simulink model "HydBrakeCU_ESP"  (Simulink 7.9)
settings: Solver=ode45  StartTime=0.0  StopTime=inf  RelTol=1e-3
PreLoadFcn:
  | HydBrakeCU_ESP_params
undefined symbols (not defined in the file or in its folder): Area_Front, Area_Rear, ay_max_off, ay_max_on, ay_per_mu_max_off, ay_per_mu_max_on, Brake_ratio, brake_valve_ctrl_kP, cat1mode1_higher, cat1mode1_lower, cat1mode2_higher, cat1mode2_lower, cat1mode3_higher, cat1mode3_lower, cat2mode1_higher, cat2mode1_lower, cat2mode2_higher, cat2mode2_lower, cat2mode3_higher, cat2mode3_lower, delta_vel, diff_lock_fac, diff_lock_off, diff_lock_on, ESP_ctrl_kD, ESP_ctrl_kI, ESP_ctrl_kP, ESP_ctrl_restore_kI, ESP_min_throttle_fac, f_ax, f_slip, g, higherlimit_highvel, higherlimit_lowvel, highervel_fac, highervelocity_fac, InitialConditionForIntegrator, limit_acc, limit_selectlow, limit_starting, limit_vdiff, locktime_throttle, lowerlimit_highvel, lowerlimit_lowvel, lowervel_fac, lowervelocity_fac, min_throttle, MPS2KMPH, MSR_ctrl_kD, MSR_ctrl_kI, MSR_ctrl_kP, MSR_min_throttle_fac, PID_kP_sideslip, PID_kP_yawrate, RADpS2RpM, rBrake, RpM2RADpS, SH_SL_switch, sideslip_vel_corr, sidesplip_deviation_max ... (+33)
libraries: CarMaker4SL x136, simulink x49, simulink_extras x6
(part 2 of 5)

== system HydBrakeCU_ESP/CarMaker/IPG Vehicle/CarAndTrailer/Forces/Tires ==
  note: The TireXX_Out signals will only be used if FileIdent is "CarMaker-Tire-CM4SL" in the tire parameter file!
      | An example parameter file can be found in Data/Tire/DT_CM4SL_UserTire.
  Sync_In : Inport
  TireFL_In : Inport  Port=2
  TireFR_In : Inport  Port=3
  TireRL_In : Inport  Port=4
  TireRR_In : Inport  Port=5
  Bus Creator{1..4} (4 alike) : BusCreator  Inputs=11
  Demux{1..3,8} (4 alike) : Demux  Outputs=7
  TireFL : Subsystem
  TireFR : Subsystem
  TireRL : Subsystem
  TireRR : Subsystem
  TireFL_Out : Outport
  TireFR_Out : Outport  Port=2
  TireRL_Out : Outport  Port=3
  TireRR_Out : Outport  Port=4
  wires:
  Sync_In/1 -> TireRR/1(Sync_In), TireRL/1(Sync_In), TireFR/1(Sync_In), TireFL/1(Sync_In)
  Bus Creator4/1 -> TireRR_Out/1
  Bus Creator2/1 -> TireRL_Out/1
  Bus Creator1/1 -> TireFR_Out/1
  Demux3/5 -> TireRR/6(Rim_turnv)  "Tire_In Rim_turnv"
  Demux3/4 -> TireRR/5(Rim_rotv)  "Tire_In Rim_rotv"
  Demux3/1 -> TireRR/2(Load)  "Tire_In Load"
  Demux3/7 -> TireRR/8(muRoad)  "Tire_In mu"
  Demux3/6 -> TireRR/7(InclinAngle)  "Tire_In Camber"
  Demux3/2 -> TireRR/3(vxtrans)  "Tire_In vxtrans"
  Demux3/3 -> TireRR/4(vytrans)  "Tire_In vytrans"
  TireRR/11(AlignTrq) -> Bus Creator4/11  "Tire_Out AlignTrq"
  TireRR/10(RollResist) -> Bus Creator4/10  "Tire_Out RollResist"
  TireRR/9(OverturnTrq) -> Bus Creator4/9  "Tire_Out OverturnTrq"
  TireRR/8(LoadFrc) -> Bus Creator4/8  "Tire_Out LoadFrc"
  TireRR/7(SideFrc) -> Bus Creator4/7  "Tire_Out SideFrc"
  TireRR/6(LongFrc) -> Bus Creator4/6  "Tire_Out LongFrc"
  TireRR/5(vBelt) -> Bus Creator4/5  "Tire_Out vBelt"
  TireRR/4(rBelt_eff) -> Bus Creator4/4  "Tire_Out rBelt_eff"
  TireRR/3(TurnSlp) -> Bus Creator4/3  "Tire_Out TurnSlp"
  TireRR/1(Slp) -> Bus Creator4/1  "Tire_Out Slp"
  TireRR/2(Alpha) -> Bus Creator4/2  "Tire_Out Alpha"
  Demux2/5 -> TireRL/6(Rim_turnv)  "Tire_In Rim_turnv"
  Demux2/4 -> TireRL/5(Rim_rotv)  "Tire_In Rim_rotv"
  Demux2/1 -> TireRL/2(Load)  "Tire_In Load"
  Demux2/7 -> TireRL/8(muRoad)  "Tire_In mu"
  Demux2/6 -> TireRL/7(InclinAngle)  "Tire_In Camber"
  Demux2/2 -> TireRL/3(vxtrans)  "Tire_In vxtrans"
  Demux2/3 -> TireRL/4(vytrans)  "Tire_In vytrans"
  TireRL/11(AlignTrq) -> Bus Creator2/11  "Tire_Out AlignTrq"
  TireRL/10(RollResist) -> Bus Creator2/10  "Tire_Out RollResist"
  TireRL/9(OverturnTrq) -> Bus Creator2/9  "Tire_Out OverturnTrq"
  TireRL/8(LoadFrc) -> Bus Creator2/8  "Tire_Out LoadFrc"
  TireRL/7(SideFrc) -> Bus Creator2/7  "Tire_Out SideFrc"
  TireRL/6(LongFrc) -> Bus Creator2/6  "Tire_Out LongFrc"
  TireRL/5(vBelt) -> Bus Creator2/5  "Tire_Out vBelt"
  TireRL/4(rBelt_eff) -> Bus Creator2/4  "Tire_Out rBelt_eff"
  TireRL/3(TurnSlp) -> Bus Creator2/3  "Tire_Out TurnSlp"
  TireRL/1(Slp) -> Bus Creator2/1  "Tire_Out Slp"
  TireRL/2(Alpha) -> Bus Creator2/2  "Tire_Out Alpha"
  Demux1/5 -> TireFR/6(Rim_turnv)  "Tire_In Rim_turnv"
  Demux1/4 -> TireFR/5(Rim_rotv)  "Tire_In Rim_rotv"
  Demux1/1 -> TireFR/2(Load)  "Tire_In Load"
  Demux1/7 -> TireFR/8(muRoad)  "Tire_In mu"
  Demux1/6 -> TireFR/7(InclinAngle)  "Tire_In Camber"
  Demux1/2 -> TireFR/3(vxtrans)  "Tire_In vxtrans"
  Demux1/3 -> TireFR/4(vytrans)  "Tire_In vytrans"
  TireFR/11(AlignTrq) -> Bus Creator1/11  "Tire_Out AlignTrq"
  TireFR/10(RollResist) -> Bus Creator1/10  "Tire_Out RollResist"
  TireFR/9(OverturnTrq) -> Bus Creator1/9  "Tire_Out OverturnTrq"
  TireFR/8(LoadFrc) -> Bus Creator1/8  "Tire_Out LoadFrc"
  TireFR/7(SideFrc) -> Bus Creator1/7  "Tire_Out SideFrc"
  TireFR/6(LongFrc) -> Bus Creator1/6  "Tire_Out LongFrc"
  TireFR/5(vBelt) -> Bus Creator1/5  "Tire_Out vBelt"
  TireFR/4(rBelt_eff) -> Bus Creator1/4  "Tire_Out rBelt_eff"
  TireFR/3(TurnSlp) -> Bus Creator1/3  "Tire_Out TurnSlp"
  TireFR/1(Slp) -> Bus Creator1/1  "Tire_Out Slp"
  TireFR/2(Alpha) -> Bus Creator1/2  "Tire_Out Alpha"
  Demux8/5 -> TireFL/6(Rim_turnv)  "Tire_In Rim_turnv"
  Demux8/4 -> TireFL/5(Rim_rotv)  "Tire_In Rim_rotv"
  TireFL_In/1 -> Demux8/1
  Demux8/1 -> TireFL/2(Load)  "Tire_In Load"
  Demux8/7 -> TireFL/8(muRoad)  "Tire_In mu"
  Demux8/6 -> TireFL/7(InclinAngle)  "Tire_In Camber"
  Demux8/2 -> TireFL/3(vxtrans)  "Tire_In vxtrans"
  Demux8/3 -> TireFL/4(vytrans)  "Tire_In vytrans"
  TireFL/11(AlignTrq) -> Bus Creator3/11  "Tire_Out AlignTrq"
  TireFL/10(RollResist) -> Bus Creator3/10  "Tire_Out RollResist"
  TireFL/9(OverturnTrq) -> Bus Creator3/9  "Tire_Out OverturnTrq"
  TireFL/8(LoadFrc) -> Bus Creator3/8  "Tire_Out LoadFrc"
  TireFL/7(SideFrc) -> Bus Creator3/7  "Tire_Out SideFrc"
  TireFL/6(LongFrc) -> Bus Creator3/6  "Tire_Out LongFrc"
  TireFL/5(vBelt) -> Bus Creator3/5  "Tire_Out vBelt"
  TireFL/4(rBelt_eff) -> Bus Creator3/4  "Tire_Out rBelt_eff"
  TireFL/3(TurnSlp) -> Bus Creator3/3  "Tire_Out TurnSlp"
  TireFL/1(Slp) -> Bus Creator3/1  "Tire_Out Slp"
  TireFL/2(Alpha) -> Bus Creator3/2  "Tire_Out Alpha"
  Bus Creator3/1 -> TireFL_Out/1
  TireFR_In/1 -> Demux1/1
  TireRL_In/1 -> Demux2/1
  TireRR_In/1 -> Demux3/1

== system HydBrakeCU_ESP/CarMaker/IPG Vehicle/CarAndTrailer/Forces/Vehicle Forces ==
  Sync_In : Inport
  Bus Creator1 : BusCreator  Inputs=12
  Bus Creator8 : BusCreator  Inputs=16
  BusCreator1 : BusCreator
  BusCreator2 : BusCreator  Inputs=9
  Demux : Demux  Outputs=16
  Demux1 : Demux  Outputs=12
  Demux2 : Demux  Outputs=13
  Forces : S-Function  FunctionName=CM_Sfun  Parameters='Forces'  EnableBusSupport=off
  Terminator : Terminator
  Sync_Out : Outport
  Car.Virtual : Outport  Port=2
  Car.Aero : Outport  Port=3
  Car.Load : Outport  Port=4
  wires:
  BusCreator1/1 -> Terminator/1  "Aero IF (in)"
  Demux2/13 -> BusCreator2/9  "car Aero Trq_1 z"
  Demux2/12 -> BusCreator2/8  "car Aero Trq_1 y"
  Demux2/11 -> BusCreator2/7  "car Aero Trq_1 x"
  Demux2/10 -> BusCreator2/6  "car Aero Frc_1 z"
  Demux2/9 -> BusCreator2/5  "car Aero Frc_1 y"
  Demux2/8 -> BusCreator2/4  "car Aero Frc_1 x"
  Demux2/7 -> BusCreator2/3  "car Aero PoA_1 z"
  Demux2/6 -> BusCreator2/2  "car Aero PoA_1 y"
  Demux2/5 -> BusCreator2/1  "car Aero PoA_1 x"
  Demux2/4 -> BusCreator1/4  "car Aero tau_1"
  Demux2/3 -> BusCreator1/3  "car Aero ApproachVel_1 z"
  Demux2/2 -> BusCreator1/2  "car Aero ApproachVel_1 y"
  Demux2/1 -> BusCreator1/1  "car Aero ApproachVel_1 x"
  Demux/16 -> Bus Creator8/16  "Car Load_3 tz"
  Demux/15 -> Bus Creator8/15  "Car Load_3 ty"
  Demux/14 -> Bus Creator8/14  "Car Load_3 tx"
  Demux/13 -> Bus Creator8/13  "Car Load_3 mass"
  Demux1/12 -> Bus Creator1/12  "Car Virtual Trq_0 z"
  Demux1/11 -> Bus Creator1/11  "Car Virtual Trq_0 y"
  Demux1/10 -> Bus Creator1/10  "Car Virtual Trq_0 x"
  Demux1/9 -> Bus Creator1/9  "Car Virtual Trq_1 z"
  Demux1/8 -> Bus Creator1/8  "Car Virtual Trq_1 y"
  Demux1/7 -> Bus Creator1/7  "Car Virtual Trq_1 x"
  Demux1/6 -> Bus Creator1/6  "Car Virtual Frc_0 z"
  Demux1/5 -> Bus Creator1/5  "Car Virtual Frc_0 y"
  Demux1/4 -> Bus Creator1/4  "Car Virtual Frc_0 x"
  Sync_In/1 -> Forces/1
  Forces/1 -> Sync_Out/1
  BusCreator2/1 -> Car.Aero/1
  Demux1/1 -> Bus Creator1/1  "Car Virtual Frc_1 x"
  Demux1/2 -> Bus Creator1/2  "Car Virtual Frc_1 y"
  Demux1/3 -> Bus Creator1/3  "Car Virtual Frc_1 z"
  Forces/3 -> Demux2/1
  Forces/2 -> Demux1/1
  Bus Creator1/1 -> Car.Virtual/1
  Bus Creator8/1 -> Car.Load/1
  Demux/1 -> Bus Creator8/1  "Car Load_0 mass"
  Demux/2 -> Bus Creator8/2  "Car Load_0 tx"
  Demux/3 -> Bus Creator8/3  "Car Load_0 ty"
  Demux/4 -> Bus Creator8/4  "Car Load_0 tz"
  Demux/5 -> Bus Creator8/5  "Car Load_1 mass"
  Demux/6 -> Bus Creator8/6  "Car Load_1 tx"
  Demux/7 -> Bus Creator8/7  "Car Load_1 ty"
  Demux/8 -> Bus Creator8/8  "Car Load_1 tz"
  Demux/9 -> Bus Creator8/9  "Car Load_2 mass"
  Demux/10 -> Bus Creator8/10  "Car Load_2 tx"
  Demux/11 -> Bus Creator8/11  "Car Load_2 ty"
  Demux/12 -> Bus Creator8/12  "Car Load_2 tz"
  Forces/4 -> Demux/1

== system HydBrakeCU_ESP/CarMaker/IPG Vehicle/CarAndTrailer/Trailer/CreateBus Car.Hitch.FrcTrq ==
  In1 : Inport
  Bus Creator7 : BusCreator  Inputs=6
  Demux7 : Demux  Outputs=6
  Out1 : Outport
  wires:
  In1/1 -> Demux7/1
  Bus Creator7/1 -> Out1/1
  Demux7/6 -> Bus Creator7/6  "Car Hitch Trq2Car z"
  Demux7/5 -> Bus Creator7/5  "Car Hitch Trq2Car y"
  Demux7/4 -> Bus Creator7/4  "Car Hitch Trq2Car x"
  Demux7/3 -> Bus Creator7/3  "Car Hitch Frc2Car z"
  Demux7/2 -> Bus Creator7/2  "Car Hitch Frc2Car y"
  Demux7/1 -> Bus Creator7/1  "Car Hitch Frc2Car x"

== system HydBrakeCU_ESP/CarMaker/IPG Vehicle/CarAndTrailer/Trailer/CreateBus Vhcl.Motion ==
  In1 : Inport
  BusCreator : BusCreator  Inputs=15
  Demux : Demux  Outputs=15
  Out1 : Outport
  wires:
  Demux/15 -> BusCreator/15  "Vhcl YawAcc"
  Demux/14 -> BusCreator/14  "Vhcl YawVel"
  Demux/13 -> BusCreator/13  "Vhcl Yaw"
  Demux/12 -> BusCreator/12  "Vhcl PitchAcc"
  Demux/11 -> BusCreator/11  "Vhcl PitchVel"
  Demux/10 -> BusCreator/10  "Vhcl Pitch"
  Demux/9 -> BusCreator/9  "Vhcl RollAcc"
  Demux/8 -> BusCreator/8  "Vhcl RollVel"
  Demux/7 -> BusCreator/7  "Vhcl Roll"
  Demux/6 -> BusCreator/6  "Vhcl Hitch_Pos z"
  Demux/5 -> BusCreator/5  "Vhcl Hitch_Pos y"
  Demux/4 -> BusCreator/4  "Vhcl Hitch_Pos x"
  Demux/3 -> BusCreator/3  "Vhcl sRoad"
  Demux/2 -> BusCreator/2  "Vhcl Distance"
  Demux/1 -> BusCreator/1  "Vhcl v"
  In1/1 -> Demux/1
  BusCreator/1 -> Out1/1

== system HydBrakeCU_ESP/CarMaker/IPG Vehicle/CarAndTrailer/Trailer/CreateBus Vhcl.PoI ==
  In1 : Inport
  Bus Creator3 : BusCreator  Inputs=18
  Demux3 : Demux  Outputs=18
  Out1 : Outport
  wires:
  Demux3/18 -> Bus Creator3/18  "Vhcl PoI_GCS Elev"
  Demux3/17 -> Bus Creator3/17  "Vhcl PoI_GCS Lat"
  Demux3/16 -> Bus Creator3/16  "Vhcl PoI_GCS Long"
  Demux3/15 -> Bus Creator3/15  "Vhcl PoI_Acc_1 z"
  Demux3/14 -> Bus Creator3/14  "Vhcl PoI_Acc_1 y"
  Demux3/13 -> Bus Creator3/13  "Vhcl PoI_Acc_1 x"
  Demux3/12 -> Bus Creator3/12  "Vhcl PoI_Vel_1 z"
  Demux3/11 -> Bus Creator3/11  "Vhcl PoI_Vel_1 y"
  Demux3/10 -> Bus Creator3/10  "Vhcl PoI_Vel_1 x"
  Demux3/9 -> Bus Creator3/9  "Vhcl PoI_Acc z"
  Demux3/8 -> Bus Creator3/8  "Vhcl PoI_Acc y"
  Demux3/7 -> Bus Creator3/7  "Vhcl PoI_Acc x"
  Demux3/6 -> Bus Creator3/6  "Vhcl PoI_Vel z"
  Demux3/5 -> Bus Creator3/5  "Vhcl PoI_Vel y"
  Demux3/4 -> Bus Creator3/4  "Vhcl PoI_Vel x"
  Demux3/3 -> Bus Creator3/3  "Vhcl PoI_Pos z"
  Demux3/2 -> Bus Creator3/2  "Vhcl PoI_Pos y"
  In1/1 -> Demux3/1
  Bus Creator3/1 -> Out1/1
  Demux3/1 -> Bus Creator3/1  "Vhcl PoI_Pos x"

== system HydBrakeCU_ESP/CarMaker/IPG Vehicle/CarAndTrailer/Trailer/CreateBus Vhcl.Steering ==
  In1 : Inport
  Bus Creator3 : BusCreator
  Demux : Demux
  Out1 : Outport
  wires:
  Bus Creator3/1 -> Out1/1
  Demux/1 -> Bus Creator3/1  "Vhcl Steering Ang"
  Demux/3 -> Bus Creator3/3  "Vhcl Steering AngAcc"
  Demux/2 -> Bus Creator3/2  "Vhcl Steering AngVel"
  Demux/4 -> Bus Creator3/4  "Vhcl Steering Trq"
  In1/1 -> Demux/1

== system HydBrakeCU_ESP/CarMaker/IPG Vehicle/CarAndTrailer/Trailer/CreateBus Vhcl.Wheel.FL ==
  In1 : Inport
  Bus Creator3 : BusCreator  Inputs=14
  Demux3 : Demux  Outputs=14
  Out1 : Outport
  wires:
  Demux3/14 -> Bus Creator3/14  "Vhcl Wheel FL Trq_WhlBearing"
  Demux3/13 -> Bus Creator3/13  "Vhcl Wheel FL Trq_T2W"
  Demux3/12 -> Bus Creator3/12  "Vhcl Wheel FL SideSlip"
  Demux3/11 -> Bus Creator3/11  "Vhcl Wheel FL LongSlip"
  Demux3/10 -> Bus Creator3/10  "Vhcl Wheel FL vBelt"
  Demux3/9 -> Bus Creator3/9  "Vhcl Wheel FL Fz"
  Demux3/8 -> Bus Creator3/8  "Vhcl Wheel FL Fy"
  Demux3/7 -> Bus Creator3/7  "Vhcl Wheel FL Fx"
  Demux3/6 -> Bus Creator3/6  "Vhcl Wheel FL r_zxy z"
  Demux3/5 -> Bus Creator3/5  "Vhcl Wheel FL r_zxy y"
  Demux3/4 -> Bus Creator3/4  "Vhcl Wheel FL r_zxy x"
  Demux3/3 -> Bus Creator3/3  "Vhcl Wheel FL t z"
  Demux3/2 -> Bus Creator3/2  "Vhcl Wheel FL t y"
  In1/1 -> Demux3/1
  Bus Creator3/1 -> Out1/1
  Demux3/1 -> Bus Creator3/1  "Vhcl Wheel FL t x"

== system HydBrakeCU_ESP/CarMaker/IPG Vehicle/CarAndTrailer/Trailer/CreateBus Vhcl.Wheel.FR ==
  In1 : Inport
  Bus Creator3 : BusCreator  Inputs=14
  Demux3 : Demux  Outputs=14
  Out1 : Outport
  wires:
  Demux3/14 -> Bus Creator3/14  "Vhcl Wheel FR Trq_WhlBearing"
  Demux3/13 -> Bus Creator3/13  "Vhcl Wheel FR Trq_T2W"
  Demux3/12 -> Bus Creator3/12  "Vhcl Wheel FR SideSlip"
  Demux3/11 -> Bus Creator3/11  "Vhcl Wheel FR LongSlip"
  Demux3/10 -> Bus Creator3/10  "Vhcl Wheel FR vBelt"
  Demux3/9 -> Bus Creator3/9  "Vhcl Wheel FR Fz"
  Demux3/8 -> Bus Creator3/8  "Vhcl Wheel FR Fy"
  Demux3/7 -> Bus Creator3/7  "Vhcl Wheel FR Fx"
  Demux3/6 -> Bus Creator3/6  "Vhcl Wheel FR r_zxy z"
  Demux3/5 -> Bus Creator3/5  "Vhcl Wheel FR r_zxy y"
  Demux3/4 -> Bus Creator3/4  "Vhcl Wheel FR r_zxy x"
  Demux3/3 -> Bus Creator3/3  "Vhcl Wheel FR t z"
  Demux3/2 -> Bus Creator3/2  "Vhcl Wheel FR t y"
  In1/1 -> Demux3/1
  Bus Creator3/1 -> Out1/1
  Demux3/1 -> Bus Creator3/1  "Vhcl Wheel FR t x"

== system HydBrakeCU_ESP/CarMaker/IPG Vehicle/CarAndTrailer/Trailer/CreateBus Vhcl.Wheel.RL ==
  In1 : Inport
  Bus Creator3 : BusCreator  Inputs=14
  Demux3 : Demux  Outputs=14
  Out1 : Outport
  wires:
  Demux3/14 -> Bus Creator3/14  "Vhcl Wheel RL Trq_WhlBearing"
  Demux3/13 -> Bus Creator3/13  "Vhcl Wheel RL Trq_T2W"
  Demux3/12 -> Bus Creator3/12  "Vhcl Wheel RL SideSlip"
  Demux3/11 -> Bus Creator3/11  "Vhcl Wheel RL LongSlip"
  Demux3/10 -> Bus Creator3/10  "Vhcl Wheel RL vBelt"
  Demux3/9 -> Bus Creator3/9  "Vhcl Wheel RL Fz"
  Demux3/8 -> Bus Creator3/8  "Vhcl Wheel RL Fy"
  Demux3/7 -> Bus Creator3/7  "Vhcl Wheel RL Fx"
  Demux3/6 -> Bus Creator3/6  "Vhcl Wheel RL r_zxy z"
  Demux3/5 -> Bus Creator3/5  "Vhcl Wheel RL r_zxy y"
  Demux3/4 -> Bus Creator3/4  "Vhcl Wheel RL r_zxy x"
  Demux3/3 -> Bus Creator3/3  "Vhcl Wheel RL t z"
  Demux3/2 -> Bus Creator3/2  "Vhcl Wheel RL t y"
  In1/1 -> Demux3/1
  Bus Creator3/1 -> Out1/1
  Demux3/1 -> Bus Creator3/1  "Vhcl Wheel RL t x"

== system HydBrakeCU_ESP/CarMaker/IPG Vehicle/CarAndTrailer/Trailer/CreateBus Vhcl.Wheel.RR ==
  In1 : Inport
  Bus Creator3 : BusCreator  Inputs=14
  Demux3 : Demux  Outputs=14
  Out1 : Outport
  wires:
  Demux3/14 -> Bus Creator3/14  "Vhcl Wheel RR Trq_WhlBearing"
  Demux3/13 -> Bus Creator3/13  "Vhcl Wheel RR Trq_T2W"
  Demux3/12 -> Bus Creator3/12  "Vhcl Wheel RR SideSlip"
  Demux3/11 -> Bus Creator3/11  "Vhcl Wheel RR LongSlip"
  Demux3/10 -> Bus Creator3/10  "Vhcl Wheel RR vBelt"
  Demux3/9 -> Bus Creator3/9  "Vhcl Wheel RR Fz"
  Demux3/8 -> Bus Creator3/8  "Vhcl Wheel RR Fy"
  Demux3/7 -> Bus Creator3/7  "Vhcl Wheel RR Fx"
  Demux3/6 -> Bus Creator3/6  "Vhcl Wheel RR r_zxy z"
  Demux3/5 -> Bus Creator3/5  "Vhcl Wheel RR r_zxy y"
  Demux3/4 -> Bus Creator3/4  "Vhcl Wheel RR r_zxy x"
  Demux3/3 -> Bus Creator3/3  "Vhcl Wheel RR t z"
  Demux3/2 -> Bus Creator3/2  "Vhcl Wheel RR t y"
  In1/1 -> Demux3/1
  Bus Creator3/1 -> Out1/1
  Demux3/1 -> Bus Creator3/1  "Vhcl Wheel RR t x"

== system HydBrakeCU_ESP/CarMaker/IPG Vehicle/Brake/HydBrakeCU Example/ESP Controller/ESP General System ==
  ESP Input Signals : Inport
  User Input Signals : Inport  Port=2
  Vehicle Input Params : Inport  Port=3
  Ideal_In : Inport  Port=4
  ABS : Subsystem
  ASR : Subsystem
  Bus Creator : BusCreator  Inputs=7
  Bus Creator2 : BusCreator  Inputs=5
  Bus Creator3 : BusCreator  Inputs=6
  Bus Creator4 : BusCreator
  ESP : Subsystem
  HSA : Subsystem
  Master Controller : Subsystem
  Signal Handling : Subsystem
  ESP Out : Outport
  wires:
  Bus Creator/1 -> ESP Out/1
  ESP Input Signals/1 -> Signal Handling/1(ESP In)
  ESP/1(ESP On) -> Master Controller/2(ESP On)  "ESP On"
  ESP/2(Pilot Valves) -> Bus Creator2/1  "Pilot Valves"
  ESP/3(Suction Valves) -> Bus Creator2/2  "Suction Valves"
  ESP/4(Brake Valves) -> Bus Creator2/3  "Brake Valves"
  ESP/5(Pump Ctrl) -> Bus Creator2/4  "Pump Ctrl"
  ESP/6(Gas_Out) -> Bus Creator2/5  "Gas_Out"
  Bus Creator2/1 -> Master Controller/3(ESP Bus)  "ESP Bus"
  ASR/1(ASR On) -> Master Controller/4(ASR On)  "ASR On"
  ABS/1(ABS On) -> Master Controller/6(ABS On)  "ABS On"
  Bus Creator3/1 -> Master Controller/5(ASR Bus)  "ASR Bus"
  Master Controller/1(ECU Flags) -> Bus Creator/1  "ECU Flags"
  Master Controller/2(Brake Valves) -> Bus Creator/2  "Brake Valves"
  Master Controller/3(Pilot Valves) -> Bus Creator/3  "Pilot Valves"
  Master Controller/4(Suction Valves) -> Bus Creator/4  "Suction Valves"
  Master Controller/5(Pump Ctrl) -> Bus Creator/5  "Pump Ctrl"
  ASR/2(Pilot Valves) -> Bus Creator3/1  "Pilot Valves"
  ASR/3(Suction Valves) -> Bus Creator3/2  "Suction Valves"
  ASR/4(Brake Valves) -> Bus Creator3/3  "Brake Valves"
  ASR/5(Pump Ctrl) -> Bus Creator3/4  "Pump Ctrl"
  ASR/6(Gas_out) -> Bus Creator3/5  "Gas_Out"
  ABS/2(Pilot Valves) -> Bus Creator4/1  "Pilot Valves"
  ABS/3(Suction Valves) -> Bus Creator4/2  "Suction Valves"
  ABS/4(Brake Valves) -> Bus Creator4/3  "Brake Valves"
  ABS/5(Pump Ctrl) -> Bus Creator4/4  "Pump Ctrl"
  Bus Creator4/1 -> Master Controller/7(ABS Bus)  "ABS Bus"
  User Input Signals/1 -> Master Controller/10(User In), ESP/4(User_In), ASR/4(User_In), ABS/4(User_In)
  Vehicle Input Params/1 -> Signal Handling/2(Vehicle Params), ESP/3(Vehicle Params), ASR/3(Vehicle Params), ABS/3(Vehicle Params)
  ASR/7(Diff_Torque) -> Bus Creator3/6  "Diff_Torque"
  Master Controller/6(Diff_Torque) -> Bus Creator/6  "Diff_Torque"
  Ideal_In/1 -> HSA/2(Ideal_In), ABS/2(Ideal_In), ESP/2(Ideal_In), ASR/2(Ideal_In)
  Master Controller/7(VC_Out) -> Bus Creator/7  "VC_Out"
  Signal Handling/2(Signal Bus ESP) -> ESP/1(ESP Signal Bus)
  Signal Handling/3(Signal Bus ASR) -> ASR/1(ASR Signal Bus)
  Signal Handling/4(Signal Bus ABS) -> ABS/1(ABS Signal Bus)
  Signal Handling/5(Signal Bus HSA) -> HSA/1(HSA Signal Bus)
  HSA/1(HSA On) -> Master Controller/8(HSA On)
  HSA/2(BrakePark_Out) -> Master Controller/9(HSA Bus)  "BrakePark"
  Signal Handling/1(Signal Bus Master Controller) -> Master Controller/1(Signal In)

== system HydBrakeCU_ESP/CarMaker/IPG Vehicle/Brake/HydBrakeCU Example/ESP Controller/ESP Input Signals ==
  HydBrakeCtrl_In : Inport
  " " : simulink_extras/Transformations/Radians to Degrees
  "   " : simulink_extras/Transformations/Radians to Degrees
  Bus Creator1 : BusCreator  Inputs=20
  Bus Selector : BusSelector  OutputSignals=Omega_B z,Acc_B y,Acc_B x
  Bus Selector1 : BusSelector  OutputSignals=HydBrakeCU pMC,HydBrakeCU pWB_FL,HydBrakeCU pWB_FR,HydBrakeCU pWB_RL,HydBrakeCU pWB_RR,HydBrakeCU Park,HydBrakeCU Pedal
  Car InertialSensor : CarMaker4SL/Car InertialSensor  xname=YRS
  Gain{,6,9..10,12..17} (10 alike) : Gain  SaturateOnIntegerOverflow=on  OutDataTypeStr=Inherit: Same as input  ParamDataTypeStr=Inherit: Same as input
  Gain{1..5,11} (6 alike) : Gain  Gain=RADpS2RpM  SaturateOnIntegerOverflow=on  OutDataTypeStr=Inherit: Same as input  ParamDataTypeStr=Inherit: Same as input
  Gain7 : Gain  Gain=1/g  SaturateOnIntegerOverflow=on  OutDataTypeStr=Inherit: Same as input  ParamDataTypeStr=Inherit: Same as input
  Gain8 : Gain  Gain=1/g  SaturateOnIntegerOverflow=on  OutDataTypeStr=Inherit: Same as input  ParamDataTypeStr=Inherit: Same as input
  Read CM Dict1 : CarMaker4SL/Read CM Dict  xname=Car.WheelSpd_FL  xsync=off
  Read CM Dict10 : CarMaker4SL/Read CM Dict  xname=PT.Clutch.rotv_out  xsync=off
  Read CM Dict11 : CarMaker4SL/Read CM Dict  xname=Steer.WhlAng  xsync=off
  Read CM Dict12 : CarMaker4SL/Read CM Dict  xname=PT.Engine.Trq  xsync=off
  Read CM Dict15 : CarMaker4SL/Read CM Dict  xname=PT.GearBox.GearNo  xsync=off
  Read CM Dict2 : CarMaker4SL/Read CM Dict  xname=Car.WheelSpd_FR  xsync=off
  Read CM Dict3 : CarMaker4SL/Read CM Dict  xname=Car.WheelSpd_RL  xsync=off
  Read CM Dict4 : CarMaker4SL/Read CM Dict  xname=Car.WheelSpd_RR  xsync=off
  Read CM Dict7 : CarMaker4SL/Read CM Dict  xname=PT.Engine.rotv  xsync=off
  Read CM Dict9 : CarMaker4SL/Read CM Dict  xname=VC.Gas  xsync=off
  Terminator : Terminator
  ESP Signals : Outport
  wires:
  Gain9/1 -> Bus Creator1/9  "Engine crankshaft output torque [Nm]"
  Gain13/1 -> Bus Creator1/14  "GearState [-]"
  " "/1 -> Bus Creator1/13  "Steering Wheel Angle [deg]"
  Gain11/1 -> Bus Creator1/12  "Torque Converter Speed [rpm]"
  Gain10/1 -> Bus Creator1/10  "Master Cylinder Pressure [bar]"
  Gain8/1 -> Bus Creator1/7  "Sensor Longitudinal acceleration [g]"
  Gain7/1 -> Bus Creator1/6  "Sensor Lateral acceleration [g]"
  "   "/1 -> Bus Creator1/5  "Sensor YawRate [degs]"
  Gain4/1 -> Bus Creator1/4  "WheelSpd RR [rpm]"
  Gain5/1 -> Bus Creator1/3  "WheelSpd RL [rpm]"
  Gain3/1 -> Bus Creator1/2  "WheelSpd FR [rpm]"
  Gain2/1 -> Bus Creator1/1  "WheelSpd FL [rpm]"
  Read CM Dict15/1 -> Gain13/1  "GearNumber [-]"
  Gain1/1 -> Bus Creator1/8  "Engine Speed [rpm]"
  Bus Selector/1 -> "   "/1  "<Omega_B z>"
  Bus Selector/3 -> Gain8/1  "<Acc_B x>"
  Car InertialSensor/2 -> Bus Selector/1
  Read CM Dict11/1 -> " "/1  "Steering Angle [rad]"
  Read CM Dict10/1 -> Gain11/1  "Clucth OutShaft [rad/s]"
  Read CM Dict9/1 -> Gain/1  "Accelerator pedal [-]"
  Bus Selector1/1 -> Gain10/1  "<HydBrakeCU pMC>"
  Read CM Dict1/1 -> Gain2/1  "WheelSpd FL [rad]/s]"
  Read CM Dict2/1 -> Gain3/1  "WheelSpd FR [rad/s]"
  Read CM Dict3/1 -> Gain5/1  "WheelSpd RL [rad/s]"
  Bus Selector/2 -> Gain7/1  "<Acc_B y>"
  Read CM Dict4/1 -> Gain4/1  "WheelSpd RR [rad/s]"
  Gain/1 -> Bus Creator1/11  "Throttle Valve Position"
  Read CM Dict12/1 -> Gain9/1  "Engine Torque [Nm]"
  Read CM Dict7/1 -> Gain1/1  "Engine RotVel [rad/s]"
  Bus Creator1/1 -> ESP Signals/1
  Bus Selector1/5 -> Gain15/1  "<HydBrakeCU pWB_RR>"
  Bus Selector1/4 -> Gain14/1  "<HydBrakeCU pWB_RL>"
  Bus Selector1/3 -> Gain12/1  "<HydBrakeCU pWB_FR>"
  Bus Selector1/2 -> Gain6/1  "<HydBrakeCU pWB_FL>"
  Gain6/1 -> Bus Creator1/15  "Cylinder Pressure FL [bar]"
  Gain12/1 -> Bus Creator1/16  "Cylinder Pressure FR [bar]"
  Gain14/1 -> Bus Creator1/17  "Cylinder Pressure RL [bar]"
  Gain15/1 -> Bus Creator1/18  "Cylinder Pressure RR [bar]"
  HydBrakeCtrl_In/1 -> Bus Selector1/1
  Car InertialSensor/1 -> Terminator/1
  Bus Selector1/6 -> Gain16/1  "<HydBrakeCU Park>"
  Gain16/1 -> Bus Creator1/19  "Park Brake Position"
  Bus Selector1/7 -> Gain17/1  "<HydBrakeCU Pedal>"
  Gain17/1 -> Bus Creator1/20  "Brake Pedal Position"

== system HydBrakeCU_ESP/CarMaker/IPG Vehicle/Brake/HydBrakeCU Example/ESP Controller/Ideal Input Signals ==
  Bus Creator1 : BusCreator  Inputs=8
  Bus Creator2 : BusCreator
  Bus Creator3 : BusCreator  Inputs=2
  Bus Creator4 : BusCreator  Inputs=2
  Bus Creator5 : BusCreator  Inputs=3
  Bus Creator6 : BusCreator  Inputs=2
  Read CM Dict1 : CarMaker4SL/Read CM Dict  xname=Car.Pitch  xsync=off
  Read CM Dict10 : CarMaker4SL/Read CM Dict  xname=Car.FzRL  xsync=off
  Read CM Dict11 : CarMaker4SL/Read CM Dict  xname=Car.YawRate  xsync=off
  Read CM Dict13 : CarMaker4SL/Read CM Dict  xname=Car.CRL.Trq_T2W  xsync=off
  Read CM Dict14 : CarMaker4SL/Read CM Dict  xname=Car.LongSlipRL  xsync=off
  Read CM Dict16 : CarMaker4SL/Read CM Dict  xname=Car.CRR.Trq_T2W  xsync=off
  Read CM Dict17 : CarMaker4SL/Read CM Dict  xname=Car.FzRR  xsync=off
  Read CM Dict19 : CarMaker4SL/Read CM Dict  xname=Car.LongSlipRR  xsync=off
  Read CM Dict2 : CarMaker4SL/Read CM Dict  xname=Car.v  xsync=off
  Read CM Dict3 : CarMaker4SL/Read CM Dict  xname=Car.muRoadFR  xsync=off
  Read CM Dict4 : CarMaker4SL/Read CM Dict  xname=Car.muRoadRL  xsync=off
  Read CM Dict5 : CarMaker4SL/Read CM Dict  xname=Car.SideSlipAngle  xsync=off
  Read CM Dict6 : CarMaker4SL/Read CM Dict  xname=Car.muRoadFL  xsync=off
  Read CM Dict7 : CarMaker4SL/Read CM Dict  xname=Car.muRoadRR  xsync=off
  Read CM Dict8 : CarMaker4SL/Read CM Dict  xname=Car.vx  xsync=off
  Read CM Dict9 : CarMaker4SL/Read CM Dict  xname=Car.vy  xsync=off
  Ideal_In : Outport
  wires:
  Read CM Dict17/1 -> Bus Creator4/2  "Ideal_FzRR"
  Read CM Dict10/1 -> Bus Creator4/1  "Ideal_FzRL"
  Read CM Dict16/1 -> Bus Creator3/2  "Ideal_Trq2WRR"
  Read CM Dict13/1 -> Bus Creator3/1  "Ideal_Trq2WRL"
  Read CM Dict6/1 -> Bus Creator2/1  "Ideal_muFL"
  Read CM Dict3/1 -> Bus Creator2/2  "Ideal_muFR"
  Read CM Dict4/1 -> Bus Creator2/3  "Ideal_muRL"
  Read CM Dict7/1 -> Bus Creator2/4  "Ideal_muRR"
  Bus Creator1/1 -> Ideal_In/1
  Read CM Dict1/1 -> Bus Creator1/1  "Ideal_Pitch"
  Read CM Dict5/1 -> Bus Creator1/3  "Ideal_SideSlipAngle"
  Read CM Dict2/1 -> Bus Creator5/1  "Ideal_Velocity"
  Read CM Dict8/1 -> Bus Creator5/2  "Ideal_Velocity_x"
  Bus Creator5/1 -> Bus Creator1/2  "Ideal_Velocity"
  Read CM Dict9/1 -> Bus Creator5/3  "Ideal_Velocity_y"
  Read CM Dict14/1 -> Bus Creator6/1  "Ideal_SlipRL"
  Read CM Dict19/1 -> Bus Creator6/2  "Ideal_SlipRR"
  Read CM Dict11/1 -> Bus Creator1/4  "Ideal_YawRate"
  Bus Creator2/1 -> Bus Creator1/5  "Ideal_mu"
  Bus Creator3/1 -> Bus Creator1/6  "Idea_Trq2W"
  Bus Creator4/1 -> Bus Creator1/7  "Ideal_Fz"
  Bus Creator6/1 -> Bus Creator1/8  "Ideal_Slip"

== system HydBrakeCU_ESP/CarMaker/IPG Vehicle/Brake/HydBrakeCU Example/ESP Controller/Output Signals ESP ==
  ESP Out : Inport
  Bus Creator : BusCreator  Inputs=6
  Bus Selector : BusSelector  OutputSignals=ECU Flags,Brake Valves,Pilot Valves,Suction Valves,Pump Ctrl,VC_Out.BrakePark,VC_Out.Brake Pedal Position,Diff_Torque,VC_Out.Load_lim
  Bus Selector1 : BusSelector  OutputSignals=ESP On,ASR On,ABS On,HSA On
  Bus Selector2 : BusSelector  OutputSignals=ASR On,MSR On,BMR On
  Bus Selector4 : BusSelector  OutputSignals=FrontDiff_Torque
  Data Type Conversion : DataTypeConversion
  Define CM Dict1 : CarMaker4SL/Define CM Dict  xname=ESP.ASR.MSR.active  xmono=off  xtype=Char  xdvaplace=VC  xnstates=2  xfirststate=0  xinitial=0
  Define CM Dict10 : CarMaker4SL/Define CM Dict  xname=ESP.ESP.active  xmono=off  xtype=Char  xdvaplace=VC  xnstates=2  xfirststate=0  xinitial=0
  Define CM Dict2 : CarMaker4SL/Define CM Dict  xname=ESP.ASR.BMR.active  xmono=off  xtype=Char  xdvaplace=VC  xnstates=2  xfirststate=0  xinitial=0
  Define CM Dict3 : CarMaker4SL/Define CM Dict  xname=ESP.ASR.active  xmono=off  xtype=Char  xdvaplace=VC  xnstates=2  xfirststate=0  xinitial=0
  Define CM Dict4 : CarMaker4SL/Define CM Dict  xname=ESP.HSA.active  xmono=off  xtype=Char  xdvaplace=VC  xnstates=2  xfirststate=0  xinitial=0
  Define CM Dict6 : CarMaker4SL/Define CM Dict  xname=ESP.ESP.lamp  xmono=off  xtype=Char  xdvaplace=VC  xnstates=2  xfirststate=0  xinitial=0
  Define CM Dict9 : CarMaker4SL/Define CM Dict  xname=ESP.ABS.Active  xmono=off  xtype=Char  xdvaplace=VC  xnstates=2  xfirststate=0  xinitial=0
  Logical Operator : Logic  Operator=OR  AllPortsSameDT=off  OutDataTypeStr=boolean
  Read CM Dict3 : CarMaker4SL/Read CM Dict  xname=ESP.User.ESP_off  xsync=off
  Write CM Dict : CarMaker4SL/Write CM Dict  xname=PT.ECU.Load_lim  xsync=off
  Write CM Dict12 : CarMaker4SL/Write CM Dict  xname=ESP.ASR.MSR.active  xsync=off
  Write CM Dict13 : CarMaker4SL/Write CM Dict  xname=ESP.ASR.BMR.active  xsync=off
  Write CM Dict15 : CarMaker4SL/Write CM Dict  xname=ESP.ASR.active  xsync=off
  Write CM Dict17 : CarMaker4SL/Write CM Dict  xname=ESP.ABS.Active  xsync=off
  Write CM Dict18 : CarMaker4SL/Write CM Dict  xname=ESP.ESP.active  xsync=off
  Write CM Dict19 : CarMaker4SL/Write CM Dict  xname=PT.Gen.DL.FDiff.DVA.Trq_A2B  xsync=off
  Write CM Dict20 : CarMaker4SL/Write CM Dict  xname=ESP.HSA.active  xsync=off
  Write CM Dict21 : CarMaker4SL/Write CM Dict  xname=ESP.ESP.lamp  xsync=off
  HydBrakeCU_Out : Outport
  wires:
  ESP Out/1 -> Bus Selector/1
  Bus Selector/1 -> Bus Selector1/1  "<ECU Flags>"
  Bus Selector1/2 -> Bus Selector2/1  "<ASR On>"
  Bus Selector1/1 -> Logical Operator/2, Write CM Dict18/1  "<ESP On>"
  Bus Selector1/3 -> Write CM Dict17/1  "<ABS On>"
  Bus Selector2/1 -> Write CM Dict15/1  "<ASR On>"
  Bus Selector2/2 -> Write CM Dict12/1  "<MSR On>"
  Bus Selector2/3 -> Write CM Dict13/1  "<BMR On>"
  Bus Selector4/1 -> Write CM Dict19/1  "<FrontDiff_Torque>"
  Bus Selector/8 -> Bus Selector4/1  "<Diff_Torque>"
  Bus Selector1/4 -> Write CM Dict20/1  "<HSA On>"
  Logical Operator/1 -> Data Type Conversion/1
  Read CM Dict3/1 -> Logical Operator/1
  Data Type Conversion/1 -> Write CM Dict21/1
  Bus Selector/2 -> Bus Creator/1  "<Brake Valves>"
  Bus Selector/3 -> Bus Creator/2  "<Pilot Valves>"
  Bus Selector/4 -> Bus Creator/3  "<Suction Valves>"
  Bus Selector/5 -> Bus Creator/4  "<Pump Ctrl>"
  Bus Creator/1 -> HydBrakeCU_Out/1
  Bus Selector/6 -> Bus Creator/5  "<BrakePark>"
  Bus Selector/9 -> Write CM Dict/1  "<Load_lim>"
  Bus Selector/7 -> Bus Creator/6  "<Brake Pedal Position>"

== system HydBrakeCU_ESP/CarMaker/IPG Vehicle/Brake/HydBrakeCU Example/ESP Controller/User Input Signals1 ==
  note: User_Drive: 1 = Front; 2 = Rear; 3 = AllWheel
  Bus Creator1 : BusCreator  Inputs=5
  Bus Creator2 : BusCreator  Inputs=5
  Bus Creator3 : BusCreator  Inputs=2
  Bus Creator4 : BusCreator  Inputs=2
  Define CM Dict1 : CarMaker4SL/Define CM Dict  xname=ESP.User.ESP_off  xmono=off  xtype=Char  xdvaplace=IO_Out  xnstates=2  xfirststate=0  xinitial=0
  Define CM Dict10 : CarMaker4SL/Define CM Dict  xname=ESP.User.HSA_off  xmono=off  xtype=Char  xdvaplace=IO_Out  xnstates=2  xfirststate=0  xinitial=0
  Define CM Dict11 : CarMaker4SL/Define CM Dict  xname=ESP.User.oneWheel_on  xmono=off  xtype=Char  xdvaplace=IO_Out  xnstates=2  xfirststate=0  xinitial=0
  Define CM Dict2 : CarMaker4SL/Define CM Dict  xname=ESP.User.ASR_off  xmono=off  xtype=Char  xdvaplace=IO_Out  xnstates=2  xfirststate=0  xinitial=0
  Define CM Dict3 : CarMaker4SL/Define CM Dict  xname=ESP.User.ABS_off  xmono=off  xtype=Char  xdvaplace=IO_Out  xnstates=2  xfirststate=0  xinitial=0
  Define CM Dict4 : CarMaker4SL/Define CM Dict  xname=ESP.User.ESP_all_off  xmono=off  xtype=Char  xdvaplace=IO_Out  xnstates=2  xfirststate=0  xinitial=0
  Define CM Dict5 : CarMaker4SL/Define CM Dict  xname=ESP.User.Drive  xmono=off  xtype=Char  xdvaplace=IO_Out  xnstates=3  xfirststate=1  xinitial=1
  Define CM Dict6 : CarMaker4SL/Define CM Dict  xname=ESP.User.SideSlip_estimator_on  xmono=off  xtype=Char  xdvaplace=IO_Out  xnstates=2  xfirststate=0  xinitial=0
  Define CM Dict7 : CarMaker4SL/Define CM Dict  xname=ESP.User.mue_estimator_on  xmono=off  xtype=Char  xdvaplace=IO_Out  xnstates=2  xfirststate=0  xinitial=0
  Define CM Dict8 : CarMaker4SL/Define CM Dict  xname=ESP.User.DiffLockDVA_on  xmono=off  xtype=Char  xdvaplace=IO_Out  xnstates=2  xfirststate=0  xinitial=0
  Define CM Dict9 : CarMaker4SL/Define CM Dict  xname=ESP.User.DiffLockDVA_Trq  xunit=Nm  xmono=off  xtype=Double4  xdvaplace=IO_Out  xnstates=2  xfirststate=0  xinitial=0
  Read CM Dict1 : CarMaker4SL/Read CM Dict  xname=ESP.User.Drive  xsync=off
  Read CM Dict10 : CarMaker4SL/Read CM Dict  xname=ESP.User.HSA_off  xsync=off
  Read CM Dict11 : CarMaker4SL/Read CM Dict  xname=ESP.User.oneWheel_on  xsync=off
  Read CM Dict2 : CarMaker4SL/Read CM Dict  xname=ESP.User.ESP_all_off  xsync=off
  Read CM Dict3 : CarMaker4SL/Read CM Dict  xname=ESP.User.ESP_off  xsync=off
  Read CM Dict4 : CarMaker4SL/Read CM Dict  xname=ESP.User.ASR_off  xsync=off
  Read CM Dict5 : CarMaker4SL/Read CM Dict  xname=ESP.User.ABS_off  xsync=off
  Read CM Dict6 : CarMaker4SL/Read CM Dict  xname=ESP.User.SideSlip_estimator_on  xsync=off
  Read CM Dict7 : CarMaker4SL/Read CM Dict  xname=ESP.User.mue_estimator_on  xsync=off
  Read CM Dict8 : CarMaker4SL/Read CM Dict  xname=ESP.User.DiffLockDVA_on  xsync=off
  Read CM Dict9 : CarMaker4SL/Read CM Dict  xname=ESP.User.DiffLockDVA_Trq  xsync=off
  User_In : Outport
  wires:
  Read CM Dict1/1 -> Bus Creator1/1  "User_Drive"
  Bus Creator1/1 -> User_In/1
  Read CM Dict5/1 -> Bus Creator2/4  "User_Switch_ABS_off"
  Read CM Dict4/1 -> Bus Creator2/3  "User_Switch_ASR_off"
  Read CM Dict3/1 -> Bus Creator2/2  "User_Switch_ESP_off"
  Read CM Dict2/1 -> Bus Creator2/1  "User_Switch_Main_off"
  Bus Creator2/1 -> Bus Creator1/2  "User_Switch"
  Read CM Dict6/1 -> Bus Creator3/1  "User_SideSlip_estimator_on"
  Read CM Dict7/1 -> Bus Creator3/2  "User_mue_estimator_on"
  Bus Creator3/1 -> Bus Creator1/3  "User_estimators_on"
  Read CM Dict8/1 -> Bus Creator4/1  "User_DiffLock_on"
  Read CM Dict9/1 -> Bus Creator4/2  "User_DiffLock_Trq"
  Bus Creator4/1 -> Bus Creator1/4  "User_DiffLock"
  Read CM Dict10/1 -> Bus Creator2/5  "User_Switch_HSA_off"
  Read CM Dict11/1 -> Bus Creator1/5  "User_oneWheel_on"

== system HydBrakeCU_ESP/CarMaker/IPG Vehicle/Brake/HydBrakeCU Example/ESP Controller/Vehicle Input Parameter ==
  note: Note:
      | We could also use
      | the left wheel as is has
      | the same coordinate
      | as regards x-axis
      | (which interests us here)
  note: Note:
      | We could also use
      | the left wheel as is has
      | the same coordinate
      | as regards x-axis
      | (which interests us here)
  Bus Creator{,1..3} (4 alike) : BusCreator
  Bus Creator4 : BusCreator  Inputs=2
  Read CM Parameter : CarMaker4SL/Read CM Parameter  xfile=TireFL  xkey=KinRollRadius  xnout=1  xdefaults=0  xmuxed=on
  Read CM Parameter1 : CarMaker4SL/Read CM Parameter  xfile=TireFR  xkey=KinRollRadius  xnout=1  xdefaults=0  xmuxed=on
  Read CM Parameter2 : CarMaker4SL/Read CM Parameter  xfile=TireRL  xkey=KinRollRadius  xnout=1  xdefaults=0  xmuxed=on
  Read CM Parameter3 : CarMaker4SL/Read CM Parameter  xfile=TireRR  xkey=KinRollRadius  xnout=1  xdefaults=0  xmuxed=on
  Read CM Parameter4 : CarMaker4SL/Read CM Parameter  xfile=Vehicle  xkey=WheelCarrier.fr.pos  xnout=1  xdefaults=0  xmuxed=on
  Read CM Parameter5 : CarMaker4SL/Read CM Parameter  xfile=Vehicle  xkey=Body.pos  xnout=1  xdefaults=0  xmuxed=on
  Read CM Parameter6 : CarMaker4SL/Read CM Parameter  xfile=Vehicle  xkey=Body.pos  xnout=1  xdefaults=0  xmuxed=on
  Read CM Parameter7 : CarMaker4SL/Read CM Parameter  xfile=Vehicle  xkey=WheelCarrier.rr.pos  xnout=1  xdefaults=0  xmuxed=on
  Read CM Parameter8 : CarMaker4SL/Read CM Parameter  xfile=Vehicle  xkey=WheelCarrier.rl.pos  xnout=2  xdefaults=0  xmuxed=off
  Read CM Parameter9 : CarMaker4SL/Read CM Parameter  xfile=Vehicle  xkey=WheelCarrier.fl.pos  xnout=2  xdefaults=0  xmuxed=off
  Steer Angle y-Data : Constant  Value=SteerAng_Out
  Steer Wheel Angle x-Data : Constant  Value=SteerWheelAng_In
  Sum3 : Sum  Inputs=+-  SaturateOnIntegerOverflow=on  InputSameDT=on  OutDataTypeStr=Inherit: Same as first input
  Sum4 : Sum  Inputs=+-  SaturateOnIntegerOverflow=on  InputSameDT=on  OutDataTypeStr=Inherit: Same as first input
  Terminator{,1..9} (10 alike) : Terminator
  z-Position of WheelCarrier FL : CarMaker4SL/Read CM Parameter  xfile=Vehicle  xkey=WheelCarrier.fl.pos  xnout=3  xdefaults=0  xmuxed=off
  z-Position of WheelCarrier FR : CarMaker4SL/Read CM Parameter  xfile=Vehicle  xkey=WheelCarrier.fr.pos  xnout=3  xdefaults=0  xmuxed=off
  z-Position of WheelCarrier RL : CarMaker4SL/Read CM Parameter  xfile=Vehicle  xkey=WheelCarrier.rl.pos  xnout=3  xdefaults=0  xmuxed=off
  z-Position of WheelCarrier RR : CarMaker4SL/Read CM Parameter  xfile=Vehicle  xkey=WheelCarrier.rr.pos  xnout=3  xdefaults=0  xmuxed=off
  Vehicle Param : Outport
  wires:
  Bus Creator1/1 -> Vehicle Param/1
  Read CM Parameter1/1 -> Bus Creator/2  "Param_RadiusFR"
  Read CM Parameter3/1 -> Bus Creator/4  "Param_RadiusRR"
  Bus Creator/1 -> Bus Creator1/1  "TireRadius"
  Read CM Parameter/1 -> Bus Creator/1  "Param_RadiusFL"
  Read CM Parameter2/1 -> Bus Creator/3  "Param_RadiusRL"
  Read CM Parameter5/1 -> Sum4/2
  Read CM Parameter4/1 -> Sum4/1
  Sum4/1 -> Bus Creator2/1  "Param_aF"
  Read CM Parameter7/1 -> Sum3/2
  Sum3/1 -> Bus Creator2/2  "Param_aR"
  Read CM Parameter6/1 -> Sum3/1
  Bus Creator2/1 -> Bus Creator1/2  "VehicleGeometry"
  Read CM Parameter8/2 -> Bus Creator2/4  "Param_bR"
  Read CM Parameter9/2 -> Bus Creator2/3  "Param_bF"
  Read CM Parameter9/1 -> Terminator/1
  Read CM Parameter8/1 -> Terminator1/1
  z-Position of WheelCarrier FL/1 -> Terminator2/1
  z-Position of WheelCarrier FL/2 -> Terminator3/1
  Bus Creator3/1 -> Bus Creator1/3  "CarrierGeometry"
  z-Position of WheelCarrier FL/3 -> Bus Creator3/1  "Param_zFL"
  z-Position of WheelCarrier FR/3 -> Bus Creator3/2  "Param_zFR"
  z-Position of WheelCarrier RL/3 -> Bus Creator3/3  "Param_zRL"
  z-Position of WheelCarrier RR/3 -> Bus Creator3/4  "Param_zRR"
  z-Position of WheelCarrier FR/1 -> Terminator4/1
  z-Position of WheelCarrier FR/2 -> Terminator5/1
  z-Position of WheelCarrier RL/1 -> Terminator6/1
  z-Position of WheelCarrier RL/2 -> Terminator7/1
  z-Position of WheelCarrier RR/1 -> Terminator8/1
  z-Position of WheelCarrier RR/2 -> Terminator9/1
  Steer Angle y-Data/1 -> Bus Creator4/2  "SteerAng_Out"
  Steer Wheel Angle x-Data/1 -> Bus Creator4/1  "SteerWheelAng_In"
  Bus Creator4/1 -> Bus Creator1/4  "SteeringGeometry"

== system HydBrakeCU_ESP/CarMaker/IPG Vehicle/Brake/HydBrakeCU Example/HydBrakeCtrl_In/CreateBus HydBrakeCU ==
  In : Inport
  BusCreator : BusCreator  Inputs=30
  Demux : Demux  Outputs=30
  Out : Outport
  wires:
  In/1 -> Demux/1
  BusCreator/1 -> Out/1
  Demux/1 -> BusCreator/1  "HydBrakeCU Pedal"
  Demux/2 -> BusCreator/2  "HydBrakeCU Park"
  Demux/3 -> BusCreator/3  "HydBrakeCU Trq_BrakeReg_max_FL"
  Demux/4 -> BusCreator/4  "HydBrakeCU Trq_BrakeReg_max_FR"
  Demux/5 -> BusCreator/5  "HydBrakeCU Trq_BrakeReg_max_RL"
  Demux/6 -> BusCreator/6  "HydBrakeCU Trq_BrakeReg_max_RR"
  Demux/7 -> BusCreator/7  "HydBrakeCU Trq_BrakeReg_FL"
  Demux/8 -> BusCreator/8  "HydBrakeCU Trq_BrakeReg_FR"
  Demux/9 -> BusCreator/9  "HydBrakeCU Trq_BrakeReg_RL"
  Demux/10 -> BusCreator/10  "HydBrakeCU Trq_BrakeReg_RR"
  Demux/11 -> BusCreator/11  "HydBrakeCU T_env"
  Demux/12 -> BusCreator/12  "HydBrakeCU Trq_WB_FL"
  Demux/13 -> BusCreator/13  "HydBrakeCU Trq_WB_FR"
  Demux/14 -> BusCreator/14  "HydBrakeCU Trq_WB_RL"
  Demux/15 -> BusCreator/15  "HydBrakeCU Trq_WB_RR"
  Demux/16 -> BusCreator/16  "HydBrakeCU Trq_PB_FL"
  Demux/17 -> BusCreator/17  "HydBrakeCU Trq_PB_FR"
  Demux/18 -> BusCreator/18  "HydBrakeCU Trq_PB_RL"
  Demux/19 -> BusCreator/19  "HydBrakeCU Trq_PB_RR"
  Demux/20 -> BusCreator/20  "HydBrakeCU Rel_SW"
  Demux/21 -> BusCreator/21  "HydBrakeCU pMC"
  Demux/22 -> BusCreator/22  "HydBrakeCU pWB_FL"
  Demux/23 -> BusCreator/23  "HydBrakeCU pWB_FR"
  Demux/24 -> BusCreator/24  "HydBrakeCU pWB_RL"
  Demux/25 -> BusCreator/25  "HydBrakeCU pWB_RR"
  Demux/26 -> BusCreator/26  "HydBrakeCU PuRetVolt"
  Demux/27 -> BusCreator/27  "HydBrakeCU PedFrc"
  Demux/28 -> BusCreator/28  "HydBrakeCU PedTravel"
  Demux/29 -> BusCreator/29  "HydBrakeCU PistTravel"
  Demux/30 -> BusCreator/30  "HydBrakeCU DiaphTravel"

== system HydBrakeCU_ESP/CarMaker/IPG Vehicle/Brake/HydBrakeCU Example/HydBrakeCtrl_In/CreateBus HydBrakeCU_Cfg ==
  In : Inport
  BusCreator : BusCreator  Inputs=3
  Demux : Demux  Outputs=3
  Out : Outport
  wires:
  In/1 -> Demux/1
  BusCreator/1 -> Out/1
  Demux/1 -> BusCreator/1  "HydBrakeCU_Cfg VhclClassId"
  Demux/2 -> BusCreator/2  "HydBrakeCU_Cfg nWheels"
  Demux/3 -> BusCreator/3  "HydBrakeCU_Cfg BrakeKind"

== system HydBrakeCU_ESP/CarMaker/IPG Vehicle/CarAndTrailer/Forces/Tires/TireFL ==
  note: Insert your tire model here.
  Sync_In : Inport
  Load : Inport  Port=2
  vxtrans : Inport  Port=3
  vytrans : Inport  Port=4
  Rim_rotv : Inport  Port=5
  Rim_turnv : Inport  Port=6
  InclinAngle : Inport  Port=7
  muRoad : Inport  Port=8
  Ground{1..11} (11 alike) : Ground
  Terminator{,1..6,12} (8 alike) : Terminator
  Slp : Outport
  Alpha : Outport  Port=2
  TurnSlp : Outport  Port=3
  rBelt_eff : Outport  Port=4
  vBelt : Outport  Port=5
  LongFrc : Outport  Port=6
  SideFrc : Outport  Port=7
  LoadFrc : Outport  Port=8
  OverturnTrq : Outport  Port=9
  RollResist : Outport  Port=10
  AlignTrq : Outport  Port=11
  wires:
  Ground11/1 -> vBelt/1
  Ground10/1 -> rBelt_eff/1
  Ground9/1 -> TurnSlp/1
  Rim_turnv/1 -> Terminator6/1
  Sync_In/1 -> Terminator12/1
  Ground2/1 -> Alpha/1
  Ground3/1 -> LongFrc/1
  Ground4/1 -> SideFrc/1
  Ground5/1 -> OverturnTrq/1
  vxtrans/1 -> Terminator1/1
  vytrans/1 -> Terminator2/1
  Rim_rotv/1 -> Terminator3/1
  InclinAngle/1 -> Terminator4/1
  muRoad/1 -> Terminator5/1
  Load/1 -> Terminator/1
  Ground1/1 -> Slp/1
  Ground6/1 -> LoadFrc/1
  Ground7/1 -> RollResist/1
  Ground8/1 -> AlignTrq/1

== system HydBrakeCU_ESP/CarMaker/IPG Vehicle/CarAndTrailer/Forces/Tires/TireFR ==
  note: Insert your tire model here.
  Sync_In : Inport
  Load : Inport  Port=2
  vxtrans : Inport  Port=3
  vytrans : Inport  Port=4
  Rim_rotv : Inport  Port=5
  Rim_turnv : Inport  Port=6
  InclinAngle : Inport  Port=7
  muRoad : Inport  Port=8
  Ground{1..11} (11 alike) : Ground
  Terminator{,1..6,12} (8 alike) : Terminator
  Slp : Outport
  Alpha : Outport  Port=2
  TurnSlp : Outport  Port=3
  rBelt_eff : Outport  Port=4
  vBelt : Outport  Port=5
  LongFrc : Outport  Port=6
  SideFrc : Outport  Port=7
  LoadFrc : Outport  Port=8
  OverturnTrq : Outport  Port=9
  RollResist : Outport  Port=10
  AlignTrq : Outport  Port=11
  wires:
  Ground11/1 -> vBelt/1
  Ground10/1 -> rBelt_eff/1
  Ground9/1 -> TurnSlp/1
  Rim_turnv/1 -> Terminator6/1
  Sync_In/1 -> Terminator12/1
  Ground2/1 -> Alpha/1
  Ground3/1 -> LongFrc/1
  Ground4/1 -> SideFrc/1
  Ground5/1 -> OverturnTrq/1
  vxtrans/1 -> Terminator1/1
  vytrans/1 -> Terminator2/1
  Rim_rotv/1 -> Terminator3/1
  InclinAngle/1 -> Terminator4/1
  muRoad/1 -> Terminator5/1
  Load/1 -> Terminator/1
  Ground1/1 -> Slp/1
  Ground6/1 -> LoadFrc/1
  Ground7/1 -> RollResist/1
  Ground8/1 -> AlignTrq/1

== system HydBrakeCU_ESP/CarMaker/IPG Vehicle/CarAndTrailer/Forces/Tires/TireRL ==
  note: Insert your tire model here.
  Sync_In : Inport
  Load : Inport  Port=2
  vxtrans : Inport  Port=3
  vytrans : Inport  Port=4
  Rim_rotv : Inport  Port=5
  Rim_turnv : Inport  Port=6
  InclinAngle : Inport  Port=7
  muRoad : Inport  Port=8
  Ground{1..11} (11 alike) : Ground
  Terminator{,1..6,12} (8 alike) : Terminator
  Slp : Outport
  Alpha : Outport  Port=2
  TurnSlp : Outport  Port=3
  rBelt_eff : Outport  Port=4
  vBelt : Outport  Port=5
  LongFrc : Outport  Port=6
  SideFrc : Outport  Port=7
  LoadFrc : Outport  Port=8
  OverturnTrq : Outport  Port=9
  RollResist : Outport  Port=10
  AlignTrq : Outport  Port=11
  wires:
  Ground11/1 -> vBelt/1
  Ground10/1 -> rBelt_eff/1
  Ground9/1 -> TurnSlp/1
  Rim_turnv/1 -> Terminator6/1
  Sync_In/1 -> Terminator12/1
  Ground2/1 -> Alpha/1
  Ground3/1 -> LongFrc/1
  Ground4/1 -> SideFrc/1
  Ground5/1 -> OverturnTrq/1
  vxtrans/1 -> Terminator1/1
  vytrans/1 -> Terminator2/1
  Rim_rotv/1 -> Terminator3/1
  InclinAngle/1 -> Terminator4/1
  muRoad/1 -> Terminator5/1
  Load/1 -> Terminator/1
  Ground1/1 -> Slp/1
  Ground6/1 -> LoadFrc/1
  Ground7/1 -> RollResist/1
  Ground8/1 -> AlignTrq/1

== system HydBrakeCU_ESP/CarMaker/IPG Vehicle/CarAndTrailer/Forces/Tires/TireRR ==
  note: Insert your tire model here.
  Sync_In : Inport
  Load : Inport  Port=2
  vxtrans : Inport  Port=3
  vytrans : Inport  Port=4
  Rim_rotv : Inport  Port=5
  Rim_turnv : Inport  Port=6
  InclinAngle : Inport  Port=7
  muRoad : Inport  Port=8
  Ground{1..11} (11 alike) : Ground
  Terminator{,1..6,12} (8 alike) : Terminator
  Slp : Outport
  Alpha : Outport  Port=2
  TurnSlp : Outport  Port=3
  rBelt_eff : Outport  Port=4
  vBelt : Outport  Port=5
  LongFrc : Outport  Port=6
  SideFrc : Outport  Port=7
  LoadFrc : Outport  Port=8
  OverturnTrq : Outport  Port=9
  RollResist : Outport  Port=10
  AlignTrq : Outport  Port=11
  wires:
  Ground11/1 -> vBelt/1
  Ground10/1 -> rBelt_eff/1
  Ground9/1 -> TurnSlp/1
  Rim_turnv/1 -> Terminator6/1
  Sync_In/1 -> Terminator12/1
  Ground2/1 -> Alpha/1
  Ground3/1 -> LongFrc/1
  Ground4/1 -> SideFrc/1
  Ground5/1 -> OverturnTrq/1
  vxtrans/1 -> Terminator1/1
  vytrans/1 -> Terminator2/1
  Rim_rotv/1 -> Terminator3/1
  InclinAngle/1 -> Terminator4/1
  muRoad/1 -> Terminator5/1
  Load/1 -> Terminator/1
  Ground1/1 -> Slp/1
  Ground6/1 -> LoadFrc/1
  Ground7/1 -> RollResist/1
  Ground8/1 -> AlignTrq/1

== system HydBrakeCU_ESP/CarMaker/IPG Vehicle/Brake/HydBrakeCU Example/ESP Controller/ESP General System/ABS ==
  note: ABS disabled when slower than v_min
  ABS Signal Bus : Inport
  Ideal_In : Inport  Port=2
  Vehicle Params : Inport  Port=3
  User_In : Inport  Port=4
  ABS ECU : Subsystem
  Bus Creator : BusCreator  Inputs=8
  Bus Creator2 : BusCreator  Inputs=2
  Bus Creator3 : BusCreator  Inputs=2
  Bus Selector3 : BusSelector  OutputSignals=ax [m/s^2],WheelSpeeds
  Bus Selector1 : BusSelector  OutputSignals=TireRadius
  Bus Selector2 : BusSelector  OutputSignals=Param_RadiusRR,Param_RadiusRL,Param_RadiusFR,Param_RadiusFL
  Bus Selector4 : BusSelector  OutputSignals=WheelSpd_RR,WheelSpd_RL,WheelSpd_FR,WheelSpd_FL
  helpsignals estimator : Subsystem
  ABS On : Outport
  Pilot Valves : Outport  Port=2
  Suction Valves : Outport  Port=3
  Brake Valves : Outport  Port=4
  Pump Ctrl : Outport  Port=5
  wires:
  helpsignals estimator/1(vref) -> ABS ECU/1(vref)
  helpsignals estimator/2(LongSlip_FL) -> ABS ECU/2(LongSlip_FL)
  helpsignals estimator/3(LongSlip_FR) -> ABS ECU/3(LongSlip_FR)
  helpsignals estimator/4(LongSlip_RL) -> ABS ECU/4(LongSlip_RL)
  ABS ECU/1(Brake Pump Ctrl) -> Pump Ctrl/1
  helpsignals estimator/5(LongSlip_RR) -> ABS ECU/5(LongSlip_RR)
  ABS ECU/10(ABS On) -> ABS On/1
  Bus Selector3/2 -> Bus Selector4/1, helpsignals estimator/4(WheelSpeeds)  "<WheelSpeeds>"
  Bus Creator/1 -> Brake Valves/1
  ABS ECU/2(Brake Valve_In_FL) -> Bus Creator/1  "Valve_In_FL"
  ABS ECU/3(Brake Valve_In_FR) -> Bus Creator/2  "Valve_In_FR"
  ABS ECU/4(Brake Valve_In_RL) -> Bus Creator/3  "Valve_In_RL"
  ABS ECU/5(Brake Valve_In_RR) -> Bus Creator/4  "Valve_In_RR"
  ABS ECU/6(Brake Valve_Out_FL) -> Bus Creator/5  "Valve_Out_FL"
  ABS ECU/7(Brake Valve_Out_FR) -> Bus Creator/6  "Valve_Out_FR"
  ABS ECU/8(Brake Valve_Out_RL) -> Bus Creator/7  "Valve_Out_RL"
  ABS ECU/9(Brake Valve_Out_RR) -> Bus Creator/8  "Valve_Out_RR"
  ABS ECU/11(Valve_PV_0) -> Bus Creator2/1  "Valve_PV_0"
  ABS ECU/12(Valve_PV_1) -> Bus Creator2/2  "Valve_PV_1"
  ABS ECU/13(Valve_SV_0) -> Bus Creator3/1  "Valve_SV_0"
  ABS ECU/14(Valve_SV_1) -> Bus Creator3/2  "Valve_SV_1"
  Bus Creator2/1 -> Pilot Valves/1
  Bus Creator3/1 -> Suction Valves/1
  User_In/1 -> helpsignals estimator/1(User_In)
  Bus Selector2/4 -> ABS ECU/10(radius_FL)  "<Param_RadiusFL>"
  Vehicle Params/1 -> Bus Selector1/1
  Bus Selector2/3 -> ABS ECU/11(radius_FR)  "<Param_RadiusFR>"
  Bus Selector2/2 -> ABS ECU/12(radius_RL)  "<Param_RadiusRL>"
  Bus Selector2/1 -> ABS ECU/13(radius_RR)  "<Param_RadiusRR>"
  Bus Selector1/1 -> Bus Selector2/1, helpsignals estimator/5(TireRadius)  "<TireRadius>"
  ABS Signal Bus/1 -> Bus Selector3/1
  Bus Selector3/1 -> helpsignals estimator/3(ax)  "<ax [m/s^2]>"
  Ideal_In/1 -> helpsignals estimator/2(Ideal_In)
  Bus Selector4/4 -> ABS ECU/6(Speed_FL)  "<WheelSpd_FL>"
  Bus Selector4/3 -> ABS ECU/7(Speed_FR)  "<WheelSpd_FR>"
  Bus Selector4/2 -> ABS ECU/8(Speed_RL)  "<WheelSpd_RL>"
  Bus Selector4/1 -> ABS ECU/9(Speed_RR)  "<WheelSpd_RR>"

== system HydBrakeCU_ESP/CarMaker/IPG Vehicle/Brake/HydBrakeCU Example/ESP Controller/ESP General System/ASR ==
  ASR Signal Bus : Inport
  Ideal_In : Inport  Port=2
  Vehicle Params : Inport  Port=3
  User_In : Inport  Port=4
  BMR ECU : Subsystem
  Bus Creator : BusCreator
  Bus Creator3 : BusCreator  Inputs=3
  Bus Selector3 : BusSelector  OutputSignals=Throttle Valve Position,WheelSpeeds
  Bus Selector : BusSelector  OutputSignals=WheelSpd_FL,WheelSpd_FR,WheelSpd_RL,WheelSpd_RR
  Bus Selector1 : BusSelector  OutputSignals=TireRadius
  Bus Selector2 : BusSelector  OutputSignals=Param_RadiusFL,Param_RadiusFR,Param_RadiusRL,Param_RadiusRR
  Constant4 : Constant  Value=MPS2KMPH
  Logical Operator2 : Logic  Operator=OR  AllPortsSameDT=off
  MSR ECU : Subsystem
  Mux1 : Mux
  Product : Product  RndMeth=Zero
  Product1 : Product  RndMeth=Zero
  ASR On : Outport
  Pilot Valves : Outport  Port=2
  Suction Valves : Outport  Port=3
  Brake Valves : Outport  Port=4
  Pump Ctrl : Outport  Port=5
  Gas_out : Outport  Port=6
  Diff_Torque : Outport  Port=7
  wires:
  Product/1 -> Product1/1
  Bus Selector/1 -> Bus Creator/1  "<WheelSpd_FL>"
  Bus Selector/2 -> Bus Creator/2  "<WheelSpd_FR>"
  Bus Selector/3 -> Bus Creator/3  "<WheelSpd_RL>"
  Bus Selector/4 -> Bus Creator/4  "<WheelSpd_RR>"
  Bus Selector2/1 -> Mux1/1  "<Param_RadiusFL>"
  MSR ECU/2(MSR On) -> Bus Creator3/1, Logical Operator2/1  "MSR On"
  BMR ECU/1(BMR On) -> Logical Operator2/2, Bus Creator3/3  "BMR On"
  BMR ECU/2(Brake Valves) -> Brake Valves/1
  Product1/1 -> BMR ECU/2(WheelVelocity [kmph]), MSR ECU/2(WheelVelocity [kmph])
  Bus Creator/1 -> Product/1
  Mux1/1 -> Product/2
  MSR ECU/1(Gas_out) -> Gas_out/1
  Bus Creator3/1 -> ASR On/1
  Logical Operator2/1 -> Bus Creator3/2  "ASR On"
  BMR ECU/3(Pilot Valves) -> Pilot Valves/1
  BMR ECU/4(Suctions Valves) -> Suction Valves/1
  BMR ECU/5(Pump Ctrl) -> Pump Ctrl/1
  User_In/1 -> MSR ECU/3(User_In), BMR ECU/3(User_In)
  BMR ECU/6(Diff_Torque) -> Diff_Torque/1  "Diff_Torque"
  Vehicle Params/1 -> Bus Selector1/1
  Bus Selector2/2 -> Mux1/2  "<Param_RadiusFR>"
  Bus Selector2/3 -> Mux1/3  "<Param_RadiusRL>"
  Bus Selector2/4 -> Mux1/4  "<Param_RadiusRR>"
  Bus Selector1/1 -> Bus Selector2/1  "<TireRadius>"
  ASR Signal Bus/1 -> Bus Selector3/1
  Bus Selector3/1 -> BMR ECU/1(Throttle), MSR ECU/1(Throttle Position)  "<Throttle Valve Position>"
  Ideal_In/1 -> MSR ECU/4(Ideal_In), BMR ECU/4(Ideal_In)
  Constant4/1 -> Product1/2
  Bus Selector3/2 -> Bus Selector/1  "<WheelSpeeds>"
